simulink model "InputOutputLinearize"  (R2013a)
settings: Solver=ode45  StartTime=0.0  StopTime=10.0  RelTol=1e-3
settings Model: Creator=Walter  LastModifiedBy=daqing_yi
settings DataIOCC: SignalLoggingSaveFormat=ModelDataLogs
settings DebuggingCC: MultiTaskDSMMsg=warning  MultiTaskCondExecSysMsg=none  StateNameClashWarn=none  StrictBusMsg=None
settings RTWCC: IncludeERTFirstTime=on

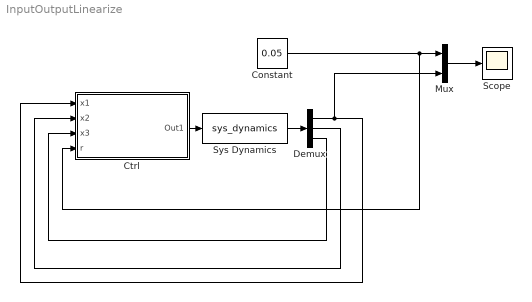
== system InputOutputLinearize ==
  Constant : Constant  Value=0.05
  "Ctrl " : Subsystem
  Demux : Demux  Outputs=3
  Mux : Mux  Inputs=2
  Scope : Scope
  Sys Dynamics : S-Function  FunctionName=sys_dynamics  EnableBusSupport=off
  wires:
  Sys Dynamics/1 -> Demux/1
  Demux/1 -> "Ctrl "/1(x1), Mux/2
  Constant/1 -> "Ctrl "/4(r), Mux/1
  Mux/1 -> Scope/1
  "Ctrl "/1(Out1) -> Sys Dynamics/1
  Demux/2 -> "Ctrl "/2(x2)
  Demux/3 -> "Ctrl "/3(x3)

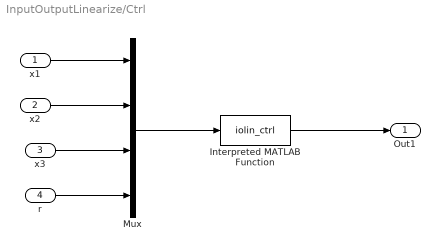
== system InputOutputLinearize/Ctrl  ==
  x1 : Inport
  x2 : Inport  Port=2
  x3 : Inport  Port=3
  r : Inport  Port=4
  Interpreted MATLAB Function : MATLABFcn  MATLABFcn=iolin_ctrl
  Mux : Mux
  Out1 : Outport
  wires:
  r/1 -> Mux/4
  x3/1 -> Mux/3
  x2/1 -> Mux/2
  x1/1 -> Mux/1
  Interpreted MATLAB Function/1 -> Out1/1
  Mux/1 -> Interpreted MATLAB Function/1
